simulink model "Controllo_Robusto"  (R2015a)
settings: Solver=ode3  StartTime=0.0  StopTime=40  FixedStep=1e-3  RelTol=1e-3
values from neighbouring files (symbols this model uses):
  alpha = in(85)    [fun_w.m]    (also in inicia_dinam.m = (BM-Bm)/(BM+Bm))
  BM = in(19)    [fun_w.m]    (also in inicia_dinam.m = norm(eval(B)))
  dif_t = in(9)    [Euler.m]    (also in rob_sic.m = 0.001)
  Kd = kd*eye(4)    [inicia_dinam.m]    (also in rob_sic.m = 50*eye(4))
  kd = in(18)    [fun_w.m]    (also in inicia_dinam.m = 100)
  Kp = kp*eye(4)    [inicia_dinam.m]    (also in rob_sic.m = 100*eye(4))
  kp = in(17)    [fun_w.m]    (also in inicia_dinam.m = 100)
  Q_vector = [Q1;Q2;Q3;Q4;Q5;Q6;Q7;Q8]    [inicia_dinam.m]
  QM = in(84)    [fun_w.m]    (also in inicia_dinam.m = norm(Q))
settings Model: Creator=TRIANOSAURIO  LastModifiedBy=TRIANOSAURIO
settings ConfigComp: CovMetricSettings=dw  CovHtmlReporting=on  CovSaveCumulativeToWorkspaceVar=on  CovSaveSingleToWorkspaceVar=on  CovExternalEMLEnable=off

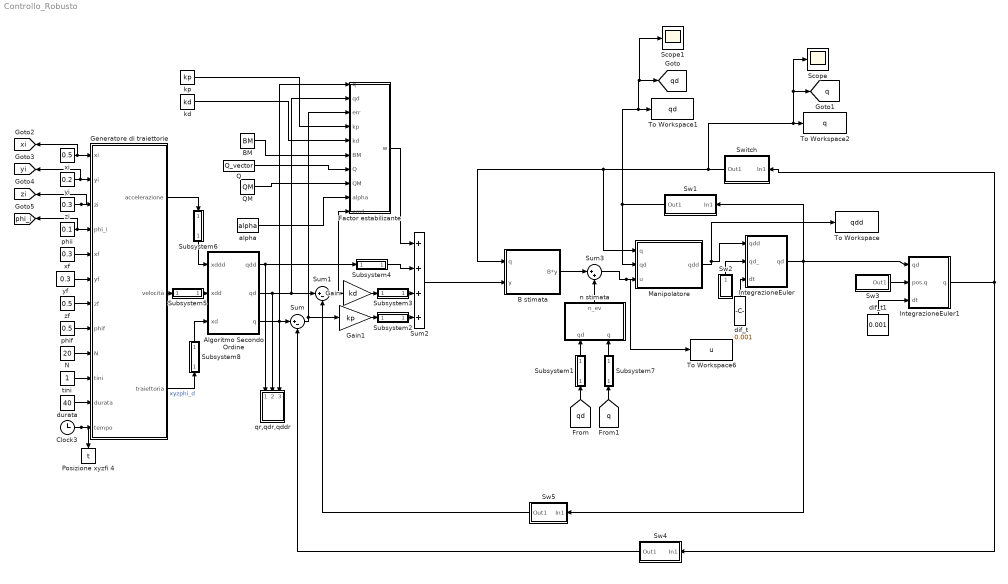
== system Controllo_Robusto ==
  Algoritmo Secondo Ordine : Subsystem
  B stimata : Subsystem
  "BM " : Constant  Value=BM
  Clock3 : Clock
  Factor estabilizante : Subsystem
  Gain : Gain  Gain=kd
  Gain1 : Gain  Gain=kp
  Generatore di traiettorie : Subsystem
  IntegrazioneEuler : Subsystem
  IntegrazioneEuler1 : Subsystem
  Manipolatore : Subsystem
  N : Constant  Value=20
  Posizione xyzfi 4 : ToWorkspace  VariableName=t  SampleTime=0.001
  Q : Constant  Value=Q_vector  VectorParams1D=off
  QM : Constant  Value=QM
  Scope : Scope
  Scope1 : Scope
  Subsystem1 : Subsystem
  Subsystem2 : Subsystem
  Subsystem3 : Subsystem
  Subsystem4 : Subsystem
  Subsystem5 : Subsystem
  Subsystem6 : Subsystem
  Subsystem7 : Subsystem
  Subsystem8 : Subsystem
  Sum : Sum  Inputs=|+-
  Sum1 : Sum  Inputs=|+-
  Sum2 : Sum  Inputs=++++
  Sum3 : Sum  Inputs=|++
  Sw1 : Subsystem
  Sw2 : Subsystem
  Sw3 : Subsystem
  Sw4 : Subsystem
  Sw5 : Subsystem
  Switch : Subsystem
  To Workspace : ToWorkspace  VariableName=qdd  SampleTime=-1
  To Workspace1 : ToWorkspace  VariableName=qd  SampleTime=-1
  To Workspace2 : ToWorkspace  VariableName=q  SampleTime=-1
  To Workspace6 : ToWorkspace  VariableName=u  SampleTime=-1
  alpha : Constant  Value=alpha
  dif_t : Constant  Value=0.001
  dif_t1 : Constant  Value=0.001
  durata : Constant  Value=40
  kd : Constant  Value=kd
  kp : Constant  Value=kp
  n stimata : Subsystem
  phif : Constant  Value=0.5
  phii : Constant  Value=0.1
  qr,qdr,qddr : Subsystem
  tini : Constant
  xf : Constant  Value=0.3
  xi : Constant  Value=0.5
  yf : Constant  Value=0.3
  yi : Constant  Value=0.2
  zf : Constant  Value=0.5
  zi : Constant  Value=0.3
  tag scope: phi_i=global, q=global, qd=global, xi=global, yi=global, zi=global
  wires:
  xi/1 -> [xi], Generatore di traiettorie/1(xi)
  yi/1 -> [yi], Generatore di traiettorie/2(yi)
  zi/1 -> [zi], Generatore di traiettorie/3(zi)
  phii/1 -> Generatore di traiettorie/4(phi_i), [phi_i]
  xf/1 -> Generatore di traiettorie/5(xf)
  yf/1 -> Generatore di traiettorie/6(yf)
  zf/1 -> Generatore di traiettorie/7(zf)
  phif/1 -> Generatore di traiettorie/8(phif)
  N/1 -> Generatore di traiettorie/9(N)
  tini/1 -> Generatore di traiettorie/10(tini)
  durata/1 -> Generatore di traiettorie/11(durata)
  Clock3/1 -> Posizione xyzfi 4/1, Generatore di traiettorie/12(tempo)
  Generatore di traiettorie/1(accelerazione) -> Subsystem6/1(In1)
  Algoritmo Secondo Ordine/3(q) -> Sum/1, Factor estabilizante/1(q), qr,qdr,qddr/3(In3)
  Sum/1 -> Factor estabilizante/3(err), Gain1/1
  Algoritmo Secondo Ordine/2(qd) -> Factor estabilizante/2(qd), Sum1/1, qr,qdr,qddr/2(In2)
  Sum1/1 -> Factor estabilizante/10(errd), Gain/1
  Algoritmo Secondo Ordine/1(qdd) -> qr,qdr,qddr/1(In1), Subsystem4/1(In1)
  Sum3/1 -> To Workspace6/1, Manipolatore/3(u)
  Manipolatore/1(qdd) -> IntegrazioneEuler/1(qdd), To Workspace/1
  Sum2/1 -> B stimata/2(y)
  B stimata/1("B*y ") -> Sum3/1
  kp/1 -> Factor estabilizante/4(kp)
  kd/1 -> Factor estabilizante/5(kd)
  "BM "/1 -> Factor estabilizante/6(BM)
  Q/1 -> Factor estabilizante/7(Q)
  QM/1 -> Factor estabilizante/8(QM)
  alpha/1 -> Factor estabilizante/9(alpha)
  Factor estabilizante/1(w) -> Sum2/1
  IntegrazioneEuler/1(qd) -> Sw5/1(In1), Sw1/1(In1), IntegrazioneEuler1/1(qd)
  IntegrazioneEuler1/1(q) -> Sw4/1(In1), Switch/1(In1)
  dif_t/1 -> IntegrazioneEuler/3(dt)
  dif_t1/1 -> IntegrazioneEuler1/3(dt)
  n stimata/1(n_ev) -> Sum3/2
  Generatore di traiettorie/3("traiettoria ") -> Subsystem8/1(In1)  "xyzphi_d"
  [qd] -> Subsystem1/1(In1)
  Subsystem1/1(Out1) -> n stimata/1(qd)
  [q] -> Subsystem7/1(In1)
  Subsystem7/1(Out1) -> n stimata/2(q)
  Gain1/1 -> Subsystem2/1(In1)
  Subsystem3/1(Out1) -> Sum2/3
  Gain/1 -> Subsystem3/1(In1)
  Subsystem2/1(Out1) -> Sum2/4
  Switch/1(Out1) -> Manipolatore/1(q), B stimata/1(q), Scope/1, [q], To Workspace2/1
  Sw1/1(Out1) -> Scope1/1, [qd], To Workspace1/1, Manipolatore/2(qd)
  Sw2/1(Out1) -> IntegrazioneEuler/2(qd_)
  Sw3/1(Out1) -> IntegrazioneEuler1/2(pos.q)
  Sw4/1(Out1) -> Sum/2
  Sw5/1(Out1) -> Sum1/2
  Subsystem4/1(Out1) -> Sum2/2
  Generatore di traiettorie/2(velocità) -> Subsystem5/1(In1)
  Subsystem5/1(Out1) -> Algoritmo Secondo Ordine/2(xdd)
  Subsystem6/1(Out1) -> Algoritmo Secondo Ordine/1(xddd)
  Subsystem8/1(Out1) -> Algoritmo Secondo Ordine/3(xd)

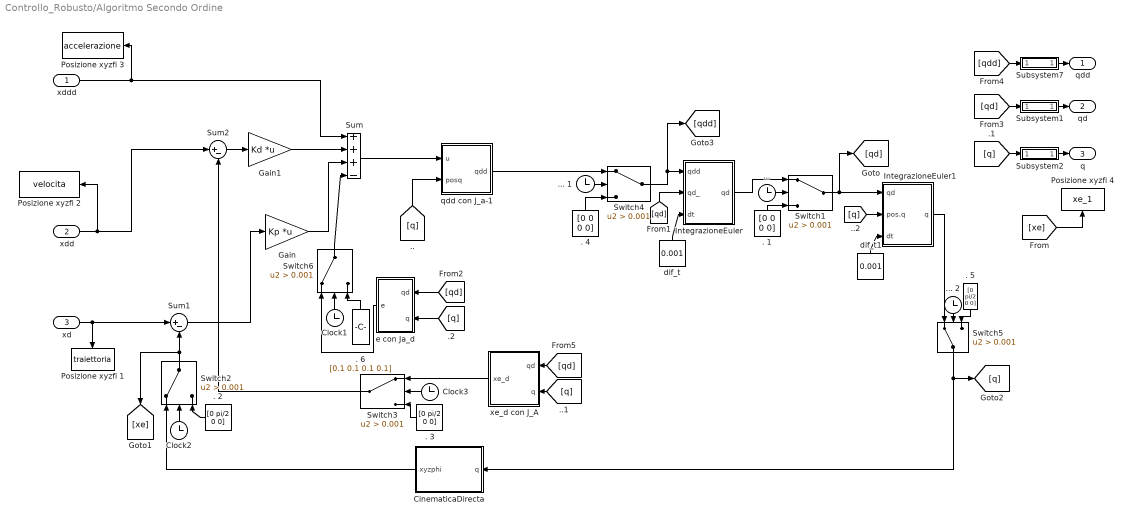
== system Controllo_Robusto/Algoritmo Secondo Ordine ==
  xddd : Inport
  xdd : Inport  Port=2
  xd : Inport  Port=3
  . 1 : Constant  Value=[0 0 0 0]
  . 2 : Constant  Value=[0 pi/2 0 0]
  . 3 : Constant  Value=[0 pi/2 0 0]
  . 4 : Constant  Value=[0 0 0 0]
  . 5 : Constant  Value=[0 pi/2 0 0]
  . 6 : Constant  Value=[0.1 0.1 0.1 0.1]
  "... " : Clock
  ... 1 : Clock
  ... 2 : Clock
  CinematicaDirecta : Subsystem
  Clock1 : Clock
  Clock2 : Clock
  Clock3 : Clock
  Gain : Gain  Gain=Kp  Multiplication=Matrix(K*u)
  Gain1 : Gain  Gain=Kd  Multiplication=Matrix(K*u)
  IntegrazioneEuler : Subsystem
  IntegrazioneEuler1 : Subsystem
  Posizione xyzfi 1 : ToWorkspace  VariableName=traiettoria  SampleTime=dif_t
  Posizione xyzfi 2 : ToWorkspace  VariableName=velocita  SampleTime=dif_t
  Posizione xyzfi 3 : ToWorkspace  VariableName=accelerazione  SampleTime=dif_t
  Posizione xyzfi 4 : ToWorkspace  VariableName=xe_1  SampleTime=dif_t
  Subsystem1 : Subsystem
  Subsystem2 : Subsystem
  Subsystem7 : Subsystem
  Sum : Sum  Inputs=+++-
  Sum1 : Sum  Inputs=|+-
  Sum2 : Sum  Inputs=|+-
  Switch{1..6} (6 alike) : Switch  Criteria=u2 > Threshold  Threshold=0.001
  dif_t : Constant  Value=0.001
  dif_t1 : Constant  Value=0.001
  e con Ja_d : Subsystem
  qdd con J_a-1 : Subsystem
  xe_d con J_A : Subsystem
  qdd : Outport
  qd : Outport  Port=2
  q : Outport  Port=3
  wires:
  Switch2/1 -> [xe], Sum1/2
  CinematicaDirecta/1(xyzphi) -> Switch2/1
  Clock2/1 -> Switch2/2
  . 2/1 -> Switch2/3
  dif_t/1 -> IntegrazioneEuler/3(dt)
  Sum1/1 -> Gain/1
  Sum/1 -> qdd con J_a-1/1(u)
  [q] -> qdd con J_a-1/2(posq)
  [qd] -> IntegrazioneEuler/2(qd_)
  xd/1 -> Sum1/1, Posizione xyzfi 1/1
  xdd/1 -> Posizione xyzfi 2/1, Sum2/1
  [q] -> xe_d con J_A/2(q)
  Gain/1 -> Sum/3
  Sum2/1 -> Gain1/1
  Gain1/1 -> Sum/2
  xddd/1 -> Posizione xyzfi 3/1, Sum/1
  Clock3/1 -> Switch3/2
  . 3/1 -> Switch3/3
  xe_d con J_A/1(xe_d) -> Switch3/1
  Switch3/1 -> Sum2/2
  dif_t1/1 -> IntegrazioneEuler1/3(dt)
  [q] -> e con Ja_d/2(q)
  [xe] -> Posizione xyzfi 4/1
  IntegrazioneEuler1/1(q) -> Switch5/1
  . 5/1 -> Switch5/3
  ... 2/1 -> Switch5/2
  Switch5/1 -> [q], CinematicaDirecta/1(q)
  [q] -> IntegrazioneEuler1/2(pos.q)
  IntegrazioneEuler/1(qd) -> Switch1/1
  . 1/1 -> Switch1/3
  "... "/1 -> Switch1/2
  Switch1/1 -> IntegrazioneEuler1/1(qd), [qd]
  [qd] -> e con Ja_d/1(qd)
  qdd con J_a-1/1(qdd) -> Switch4/1
  . 4/1 -> Switch4/3
  ... 1/1 -> Switch4/2
  Switch4/1 -> [qdd], IntegrazioneEuler/1(qdd)
  [qd] -> xe_d con J_A/1(qd)
  Clock1/1 -> Switch6/2
  . 6/1 -> Switch6/3
  e con Ja_d/1(e) -> Switch6/1
  Switch6/1 -> Sum/4
  [qdd] -> Subsystem7/1(In1)
  [qd] -> Subsystem1/1(In1)
  Subsystem1/1(Out1) -> qd/1
  [q] -> Subsystem2/1(In1)
  Subsystem2/1(Out1) -> q/1
  Subsystem7/1(Out1) -> qdd/1

== system Controllo_Robusto/B stimata ==
  q : Inport
  y : Inport  Port=2
  "B_stimata " : MATLABFcn  MATLABFcn=fun_B
  Mux1 : Mux  Inputs=2
  "B*y " : Outport
  wires:
  "B_stimata "/1 -> "B*y "/1
  Mux1/1 -> "B_stimata "/1
  q/1 -> Mux1/2
  y/1 -> Mux1/1

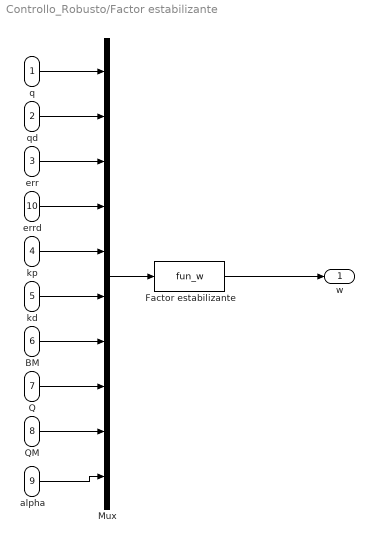
== system Controllo_Robusto/Factor estabilizante ==
  q : Inport
  qd : Inport  Port=2
  err : Inport  Port=3
  kp : Inport  Port=4
  kd : Inport  Port=5
  BM : Inport  Port=6
  Q : Inport  Port=7
  QM : Inport  Port=8
  alpha : Inport  Port=9
  errd : Inport  Port=10
  Factor estabilizante : MATLABFcn  MATLABFcn=fun_w  OutputDimensions=4
  Mux : Mux  Inputs=10
  w : Outport
  wires:
  Mux/1 -> Factor estabilizante/1
  qd/1 -> Mux/2
  q/1 -> Mux/1
  err/1 -> Mux/3
  errd/1 -> Mux/4
  kp/1 -> Mux/5
  kd/1 -> Mux/6
  BM/1 -> Mux/7
  Q/1 -> Mux/8
  QM/1 -> Mux/9
  alpha/1 -> Mux/10
  Factor estabilizante/1 -> w/1

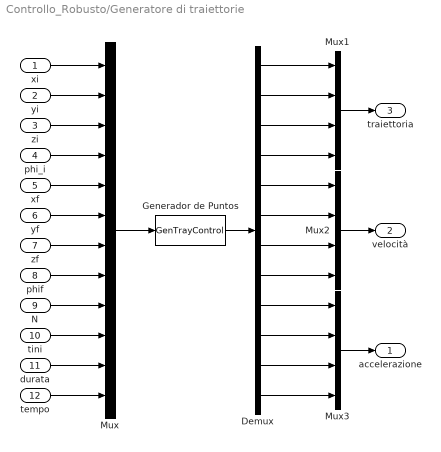
== system Controllo_Robusto/Generatore di traiettorie ==
  xi : Inport
  yi : Inport  Port=2
  zi : Inport  Port=3
  phi_i : Inport  Port=4
  xf : Inport  Port=5
  yf : Inport  Port=6
  zf : Inport  Port=7
  phif : Inport  Port=8
  N : Inport  Port=9
  tini : Inport  Port=10
  durata : Inport  Port=11
  tempo : Inport  Port=12
  Demux : Demux  Outputs=12
  Generador de Puntos : MATLABFcn  MATLABFcn=GenTrayControl  OutputDimensions=12
  Mux : Mux  Inputs=12
  Mux1 : Mux
  Mux2 : Mux
  Mux3 : Mux
  accelerazione : Outport
  velocità : Outport  Port=2
  "traiettoria " : Outport  Port=3
  wires:
  Mux/1 -> Generador de Puntos/1
  xi/1 -> Mux/1
  yi/1 -> Mux/2
  zi/1 -> Mux/3
  phi_i/1 -> Mux/4
  xf/1 -> Mux/5
  yf/1 -> Mux/6
  zf/1 -> Mux/7
  phif/1 -> Mux/8
  N/1 -> Mux/9
  tini/1 -> Mux/10
  durata/1 -> Mux/11
  tempo/1 -> Mux/12
  Generador de Puntos/1 -> Demux/1
  Mux1/1 -> "traiettoria "/1
  Mux2/1 -> velocità/1
  Mux3/1 -> accelerazione/1
  Demux/12 -> Mux3/4
  Demux/11 -> Mux3/3
  Demux/10 -> Mux3/2
  Demux/9 -> Mux3/1
  Demux/8 -> Mux2/4
  Demux/7 -> Mux2/3
  Demux/6 -> Mux2/2
  Demux/5 -> Mux2/1
  Demux/4 -> Mux1/4
  Demux/1 -> Mux1/1
  Demux/2 -> Mux1/2
  Demux/3 -> Mux1/3

== system Controllo_Robusto/IntegrazioneEuler ==
  qdd : Inport
  qd_ : Inport  Port=2
  dt : Inport  Port=3
  Euler : MATLABFcn  MATLABFcn=Euler  OutputDimensions=4
  Mux2 : Mux  Inputs=3
  Subsystem4 : Subsystem
  qd : Outport
  wires:
  Euler/1 -> Subsystem4/1(In1)
  qdd/1 -> Mux2/1
  Mux2/1 -> Euler/1
  qd_/1 -> Mux2/2
  dt/1 -> Mux2/3
  Subsystem4/1(Out1) -> qd/1

== system Controllo_Robusto/IntegrazioneEuler1 ==
  qd : Inport
  pos.q : Inport  Port=2
  dt : Inport  Port=3
  Euler : MATLABFcn  MATLABFcn=Euler  OutputDimensions=4
  Mux2 : Mux  Inputs=3
  Subsystem4 : Subsystem
  q : Outport
  wires:
  dt/1 -> Mux2/3
  pos.q/1 -> Mux2/2
  Mux2/1 -> Euler/1
  qd/1 -> Mux2/1
  Euler/1 -> Subsystem4/1(In1)
  Subsystem4/1(Out1) -> q/1

== system Controllo_Robusto/Manipolatore ==
  q : Inport
  qd : Inport  Port=2
  u : Inport  Port=3
  Manipolatore : MATLABFcn  MATLABFcn=modelo_dinam  OutputDimensions=4
  Mux3 : Mux
  Subsystem4 : Subsystem
  qdd : Outport
  wires:
  Mux3/1 -> Manipolatore/1
  u/1 -> Mux3/1
  q/1 -> Mux3/2
  qd/1 -> Mux3/3
  Manipolatore/1 -> Subsystem4/1(In1)
  Subsystem4/1(Out1) -> Mux3/4, qdd/1

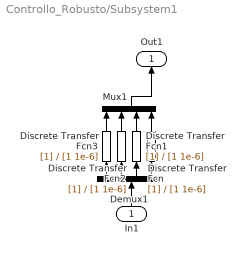
== system Controllo_Robusto/Subsystem1 ==
  In1 : Inport
  Demux1 : Demux
  Discrete Transfer Fcn{,1..3} (4 alike) : DiscreteTransferFcn  Denominator=[1 1e-6]  SampleTime=0.001
  Mux1 : Mux
  Out1 : Outport
  wires:
  In1/1 -> Demux1/1
  Mux1/1 -> Out1/1
  Discrete Transfer Fcn/1 -> Mux1/4
  Demux1/4 -> Discrete Transfer Fcn/1
  Discrete Transfer Fcn1/1 -> Mux1/3
  Demux1/3 -> Discrete Transfer Fcn1/1
  Discrete Transfer Fcn2/1 -> Mux1/2
  Demux1/2 -> Discrete Transfer Fcn2/1
  Discrete Transfer Fcn3/1 -> Mux1/1
  Demux1/1 -> Discrete Transfer Fcn3/1

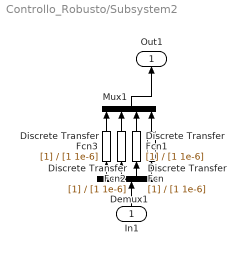
== system Controllo_Robusto/Subsystem2 ==
  In1 : Inport
  Demux1 : Demux
  Discrete Transfer Fcn{,1..3} (4 alike) : DiscreteTransferFcn  Denominator=[1 1e-6]  SampleTime=0.001
  Mux1 : Mux
  Out1 : Outport
  wires:
  In1/1 -> Demux1/1
  Mux1/1 -> Out1/1
  Discrete Transfer Fcn/1 -> Mux1/4
  Demux1/4 -> Discrete Transfer Fcn/1
  Discrete Transfer Fcn1/1 -> Mux1/3
  Demux1/3 -> Discrete Transfer Fcn1/1
  Discrete Transfer Fcn2/1 -> Mux1/2
  Demux1/2 -> Discrete Transfer Fcn2/1
  Discrete Transfer Fcn3/1 -> Mux1/1
  Demux1/1 -> Discrete Transfer Fcn3/1

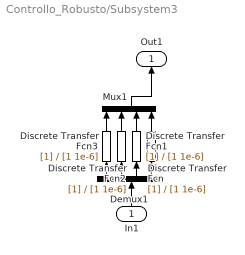
== system Controllo_Robusto/Subsystem3 ==
  In1 : Inport
  Demux1 : Demux
  Discrete Transfer Fcn{,1..3} (4 alike) : DiscreteTransferFcn  Denominator=[1 1e-6]  SampleTime=0.001
  Mux1 : Mux
  Out1 : Outport
  wires:
  Demux1/1 -> Discrete Transfer Fcn3/1
  Discrete Transfer Fcn3/1 -> Mux1/1
  Demux1/2 -> Discrete Transfer Fcn2/1
  Discrete Transfer Fcn2/1 -> Mux1/2
  Demux1/3 -> Discrete Transfer Fcn1/1
  Discrete Transfer Fcn1/1 -> Mux1/3
  Demux1/4 -> Discrete Transfer Fcn/1
  Discrete Transfer Fcn/1 -> Mux1/4
  Mux1/1 -> Out1/1
  In1/1 -> Demux1/1

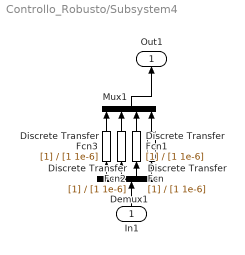
== system Controllo_Robusto/Subsystem4 ==
  In1 : Inport
  Demux1 : Demux
  Discrete Transfer Fcn{,1..3} (4 alike) : DiscreteTransferFcn  Denominator=[1 1e-6]  SampleTime=0.001
  Mux1 : Mux
  Out1 : Outport
  wires:
  In1/1 -> Demux1/1
  Mux1/1 -> Out1/1
  Discrete Transfer Fcn/1 -> Mux1/4
  Demux1/4 -> Discrete Transfer Fcn/1
  Discrete Transfer Fcn1/1 -> Mux1/3
  Demux1/3 -> Discrete Transfer Fcn1/1
  Discrete Transfer Fcn2/1 -> Mux1/2
  Demux1/2 -> Discrete Transfer Fcn2/1
  Discrete Transfer Fcn3/1 -> Mux1/1
  Demux1/1 -> Discrete Transfer Fcn3/1

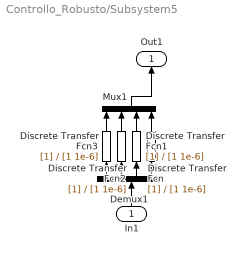
== system Controllo_Robusto/Subsystem5 ==
  In1 : Inport
  Demux1 : Demux
  Discrete Transfer Fcn{,1..3} (4 alike) : DiscreteTransferFcn  Denominator=[1 1e-6]  SampleTime=0.001
  Mux1 : Mux
  Out1 : Outport
  wires:
  In1/1 -> Demux1/1
  Mux1/1 -> Out1/1
  Discrete Transfer Fcn/1 -> Mux1/4
  Demux1/4 -> Discrete Transfer Fcn/1
  Discrete Transfer Fcn1/1 -> Mux1/3
  Demux1/3 -> Discrete Transfer Fcn1/1
  Discrete Transfer Fcn2/1 -> Mux1/2
  Demux1/2 -> Discrete Transfer Fcn2/1
  Discrete Transfer Fcn3/1 -> Mux1/1
  Demux1/1 -> Discrete Transfer Fcn3/1

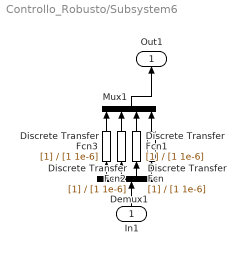
== system Controllo_Robusto/Subsystem6 ==
  In1 : Inport
  Demux1 : Demux
  Discrete Transfer Fcn{,1..3} (4 alike) : DiscreteTransferFcn  Denominator=[1 1e-6]  SampleTime=0.001
  Mux1 : Mux
  Out1 : Outport
  wires:
  Demux1/1 -> Discrete Transfer Fcn3/1
  Discrete Transfer Fcn3/1 -> Mux1/1
  Demux1/2 -> Discrete Transfer Fcn2/1
  Discrete Transfer Fcn2/1 -> Mux1/2
  Demux1/3 -> Discrete Transfer Fcn1/1
  Discrete Transfer Fcn1/1 -> Mux1/3
  Demux1/4 -> Discrete Transfer Fcn/1
  Discrete Transfer Fcn/1 -> Mux1/4
  Mux1/1 -> Out1/1
  In1/1 -> Demux1/1

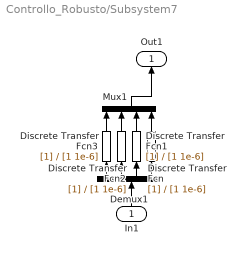
== system Controllo_Robusto/Subsystem7 ==
  In1 : Inport
  Demux1 : Demux
  Discrete Transfer Fcn{,1..3} (4 alike) : DiscreteTransferFcn  Denominator=[1 1e-6]  SampleTime=0.001
  Mux1 : Mux
  Out1 : Outport
  wires:
  In1/1 -> Demux1/1
  Mux1/1 -> Out1/1
  Discrete Transfer Fcn/1 -> Mux1/4
  Demux1/4 -> Discrete Transfer Fcn/1
  Discrete Transfer Fcn1/1 -> Mux1/3
  Demux1/3 -> Discrete Transfer Fcn1/1
  Discrete Transfer Fcn2/1 -> Mux1/2
  Demux1/2 -> Discrete Transfer Fcn2/1
  Discrete Transfer Fcn3/1 -> Mux1/1
  Demux1/1 -> Discrete Transfer Fcn3/1

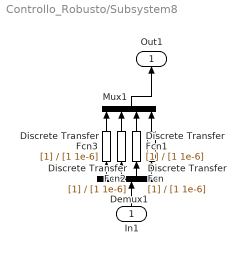
== system Controllo_Robusto/Subsystem8 ==
  In1 : Inport
  Demux1 : Demux
  Discrete Transfer Fcn{,1..3} (4 alike) : DiscreteTransferFcn  Denominator=[1 1e-6]  SampleTime=0.001
  Mux1 : Mux
  Out1 : Outport
  wires:
  In1/1 -> Demux1/1
  Mux1/1 -> Out1/1
  Discrete Transfer Fcn/1 -> Mux1/4
  Demux1/4 -> Discrete Transfer Fcn/1
  Discrete Transfer Fcn1/1 -> Mux1/3
  Demux1/3 -> Discrete Transfer Fcn1/1
  Discrete Transfer Fcn2/1 -> Mux1/2
  Demux1/2 -> Discrete Transfer Fcn2/1
  Discrete Transfer Fcn3/1 -> Mux1/1
  Demux1/1 -> Discrete Transfer Fcn3/1

== system Controllo_Robusto/Sw1 ==
  In1 : Inport
  . 5 : Constant  Value=[0 0 0 0]
  Clock6 : Clock
  Subsystem9 : Subsystem
  Switch5 : Switch  Criteria=u2 > Threshold  Threshold=0.001
  Out1 : Outport
  wires:
  In1/1 -> Subsystem9/1(In1)
  Subsystem9/1(Out1) -> Switch5/1
  Switch5/1 -> Out1/1
  . 5/1 -> Switch5/3
  Clock6/1 -> Switch5/2

== system Controllo_Robusto/Sw2 ==
  . 7 : Constant  Value=[0 pi/2 0 0]
  "... " : Clock
  Switch7 : Switch  Criteria=u2 > Threshold  Threshold=0.001
  Out1 : Outport
  wires:
  "... "/1 -> Switch7/2
  . 7/1 -> Switch7/3
  [qd] -> Switch7/1
  Switch7/1 -> Out1/1

== system Controllo_Robusto/Sw3 ==
  ... 1 : Clock
  Switch8 : Switch  Criteria=u2 > Threshold  Threshold=0.001
  dif_t : Constant  Value=[0 pi/2 0 0]
  Out1 : Outport
  wires:
  [q] -> Switch8/1
  dif_t/1 -> Switch8/3
  Switch8/1 -> Out1/1
  ... 1/1 -> Switch8/2

== system Controllo_Robusto/Sw4 ==
  In1 : Inport
  Clock1 : Clock
  Switch3 : Switch  Criteria=u2 > Threshold  Threshold=0.001
  dif_t : Constant  Value=[0 pi/2 0 0]
  Out1 : Outport
  wires:
  In1/1 -> Switch3/1
  dif_t/1 -> Switch3/3
  Clock1/1 -> Switch3/2
  Switch3/1 -> Out1/1

== system Controllo_Robusto/Sw5 ==
  In1 : Inport
  . 1 : Constant  Value=[0 0 0 0]
  Clock2 : Clock
  Subsystem4 : Subsystem
  Switch1 : Switch  Criteria=u2 > Threshold  Threshold=0.001
  Out1 : Outport
  wires:
  In1/1 -> Subsystem4/1(In1)
  Clock2/1 -> Switch1/2
  . 1/1 -> Switch1/3
  Switch1/1 -> Out1/1
  Subsystem4/1(Out1) -> Switch1/1

== system Controllo_Robusto/Switch ==
  In1 : Inport
  Clock7 : Clock
  Subsystem8 : Subsystem
  Switch6 : Switch  Criteria=u2 > Threshold  Threshold=0.001
  dif_t : Constant  Value=[0 pi/2 0 0]
  Out1 : Outport
  wires:
  In1/1 -> Subsystem8/1(In1)
  Subsystem8/1(Out1) -> Switch6/1
  Clock7/1 -> Switch6/2
  Switch6/1 -> Out1/1
  dif_t/1 -> Switch6/3

== system Controllo_Robusto/n stimata ==
  qd : Inport
  q : Inport  Port=2
  Mux2 : Mux  Inputs=2
  "n_stimata " : MATLABFcn  MATLABFcn=fun_n  OutputDimensions=4
  n_ev : Outport
  wires:
  Mux2/1 -> "n_stimata "/1
  q/1 -> Mux2/1
  qd/1 -> Mux2/2
  "n_stimata "/1 -> n_ev/1

== system Controllo_Robusto/qr,qdr,qddr ==
  In1 : Inport
  In2 : Inport  Port=2
  In3 : Inport  Port=3
  To Workspace3 : ToWorkspace  VariableName=qr  SampleTime=-1
  To Workspace4 : ToWorkspace  VariableName=qdr  SampleTime=-1
  To Workspace5 : ToWorkspace  VariableName=qddr  SampleTime=-1
  wires:
  In3/1 -> To Workspace3/1
  In2/1 -> To Workspace4/1
  In1/1 -> To Workspace5/1

== system Controllo_Robusto/Algoritmo Secondo Ordine/CinematicaDirecta ==
  q : Inport
  Interpreted MATLAB Function : MATLABFcn  MATLABFcn=CinematicaDirecta
  xyzphi : Outport
  wires:
  q/1 -> Interpreted MATLAB Function/1
  Interpreted MATLAB Function/1 -> xyzphi/1

== system Controllo_Robusto/Algoritmo Secondo Ordine/IntegrazioneEuler ==
  qdd : Inport
  qd_ : Inport  Port=2
  dt : Inport  Port=3
  Euler : MATLABFcn  MATLABFcn=Euler
  Mux2 : Mux  Inputs=3
  qd : Outport
  wires:
  Euler/1 -> qd/1
  qdd/1 -> Mux2/1
  Mux2/1 -> Euler/1
  qd_/1 -> Mux2/2
  dt/1 -> Mux2/3

== system Controllo_Robusto/Algoritmo Secondo Ordine/IntegrazioneEuler1 ==
  qd : Inport
  pos.q : Inport  Port=2
  dt : Inport  Port=3
  Euler : MATLABFcn  MATLABFcn=Euler
  Mux2 : Mux  Inputs=3
  q : Outport
  wires:
  dt/1 -> Mux2/3
  pos.q/1 -> Mux2/2
  Mux2/1 -> Euler/1
  qd/1 -> Mux2/1
  Euler/1 -> q/1

== system Controllo_Robusto/Algoritmo Secondo Ordine/Subsystem1 ==
  In1 : Inport
  Demux1 : Demux
  Discrete Transfer Fcn{,1..3} (4 alike) : DiscreteTransferFcn  Denominator=[1 1e-6]  SampleTime=0.001
  Mux1 : Mux
  Out1 : Outport
  wires:
  Demux1/1 -> Discrete Transfer Fcn3/1
  Discrete Transfer Fcn3/1 -> Mux1/1
  Demux1/2 -> Discrete Transfer Fcn2/1
  Discrete Transfer Fcn2/1 -> Mux1/2
  Demux1/3 -> Discrete Transfer Fcn1/1
  Discrete Transfer Fcn1/1 -> Mux1/3
  Demux1/4 -> Discrete Transfer Fcn/1
  Discrete Transfer Fcn/1 -> Mux1/4
  Mux1/1 -> Out1/1
  In1/1 -> Demux1/1

== system Controllo_Robusto/Algoritmo Secondo Ordine/Subsystem2 ==
  In1 : Inport
  Demux1 : Demux
  Discrete Transfer Fcn{,1..3} (4 alike) : DiscreteTransferFcn  Denominator=[1 1e-6]  SampleTime=0.001
  Mux1 : Mux
  Out1 : Outport
  wires:
  In1/1 -> Demux1/1
  Mux1/1 -> Out1/1
  Discrete Transfer Fcn/1 -> Mux1/4
  Demux1/4 -> Discrete Transfer Fcn/1
  Discrete Transfer Fcn1/1 -> Mux1/3
  Demux1/3 -> Discrete Transfer Fcn1/1
  Discrete Transfer Fcn2/1 -> Mux1/2
  Demux1/2 -> Discrete Transfer Fcn2/1
  Discrete Transfer Fcn3/1 -> Mux1/1
  Demux1/1 -> Discrete Transfer Fcn3/1

== system Controllo_Robusto/Algoritmo Secondo Ordine/Subsystem7 ==
  In1 : Inport
  Demux1 : Demux
  Discrete Transfer Fcn{,1..3} (4 alike) : DiscreteTransferFcn  Denominator=[1 1e-6]  SampleTime=0.001
  Mux1 : Mux
  Out1 : Outport
  wires:
  In1/1 -> Demux1/1
  Mux1/1 -> Out1/1
  Discrete Transfer Fcn/1 -> Mux1/4
  Demux1/4 -> Discrete Transfer Fcn/1
  Discrete Transfer Fcn1/1 -> Mux1/3
  Demux1/3 -> Discrete Transfer Fcn1/1
  Discrete Transfer Fcn2/1 -> Mux1/2
  Demux1/2 -> Discrete Transfer Fcn2/1
  Discrete Transfer Fcn3/1 -> Mux1/1
  Demux1/1 -> Discrete Transfer Fcn3/1

== system Controllo_Robusto/Algoritmo Secondo Ordine/e con Ja_d ==
  qd : Inport
  q : Inport  Port=2
  JacobianaDerivada : MATLABFcn  MATLABFcn=JacobianaDerivada
  Mux2 : Mux  Inputs=2
  Subsystem4 : Subsystem
  e : Outport
  wires:
  q/1 -> Mux2/2
  JacobianaDerivada/1 -> Subsystem4/1(In1)
  qd/1 -> Mux2/1
  Mux2/1 -> JacobianaDerivada/1
  Subsystem4/1(Out1) -> e/1

== system Controllo_Robusto/Algoritmo Secondo Ordine/qdd con J_a-1 ==
  u : Inport
  posq : Inport  Port=2
  Mux2 : Mux  Inputs=2
  qd_mediante_Ja-1 : MATLABFcn  MATLABFcn=JacobianaNumerica
  qdd : Outport
  wires:
  qd_mediante_Ja-1/1 -> qdd/1
  Mux2/1 -> qd_mediante_Ja-1/1
  u/1 -> Mux2/1
  posq/1 -> Mux2/2

== system Controllo_Robusto/Algoritmo Secondo Ordine/xe_d con J_A ==
  qd : Inport
  q : Inport  Port=2
  Mux2 : Mux  Inputs=2
  "xe^{.}" : MATLABFcn  MATLABFcn=JacobianaAnalitica
  xe_d : Outport
  wires:
  q/1 -> Mux2/2
  Mux2/1 -> "xe^{.}"/1
  qd/1 -> Mux2/1
  "xe^{.}"/1 -> xe_d/1

== system Controllo_Robusto/IntegrazioneEuler/Subsystem4 ==
  In1 : Inport
  Demux1 : Demux
  Discrete Transfer Fcn{,1..3} (4 alike) : DiscreteTransferFcn  Denominator=[1 1e-6]  SampleTime=0.001
  Mux1 : Mux
  Out1 : Outport
  wires:
  In1/1 -> Demux1/1
  Mux1/1 -> Out1/1
  Discrete Transfer Fcn/1 -> Mux1/4
  Demux1/4 -> Discrete Transfer Fcn/1
  Discrete Transfer Fcn1/1 -> Mux1/3
  Demux1/3 -> Discrete Transfer Fcn1/1
  Discrete Transfer Fcn2/1 -> Mux1/2
  Demux1/2 -> Discrete Transfer Fcn2/1
  Discrete Transfer Fcn3/1 -> Mux1/1
  Demux1/1 -> Discrete Transfer Fcn3/1

== system Controllo_Robusto/IntegrazioneEuler1/Subsystem4 ==
  In1 : Inport
  Demux1 : Demux
  Discrete Transfer Fcn{,1..3} (4 alike) : DiscreteTransferFcn  Denominator=[1 1e-6]  SampleTime=0.001
  Mux1 : Mux
  Out1 : Outport
  wires:
  In1/1 -> Demux1/1
  Mux1/1 -> Out1/1
  Discrete Transfer Fcn/1 -> Mux1/4
  Demux1/4 -> Discrete Transfer Fcn/1
  Discrete Transfer Fcn1/1 -> Mux1/3
  Demux1/3 -> Discrete Transfer Fcn1/1
  Discrete Transfer Fcn2/1 -> Mux1/2
  Demux1/2 -> Discrete Transfer Fcn2/1
  Discrete Transfer Fcn3/1 -> Mux1/1
  Demux1/1 -> Discrete Transfer Fcn3/1

== system Controllo_Robusto/Manipolatore/Subsystem4 ==
  In1 : Inport
  Demux1 : Demux
  Discrete Transfer Fcn{,1..3} (4 alike) : DiscreteTransferFcn  Denominator=[1 1e-6]  SampleTime=0.001
  Mux1 : Mux
  Out1 : Outport
  wires:
  In1/1 -> Demux1/1
  Mux1/1 -> Out1/1
  Discrete Transfer Fcn/1 -> Mux1/4
  Demux1/4 -> Discrete Transfer Fcn/1
  Discrete Transfer Fcn1/1 -> Mux1/3
  Demux1/3 -> Discrete Transfer Fcn1/1
  Discrete Transfer Fcn2/1 -> Mux1/2
  Demux1/2 -> Discrete Transfer Fcn2/1
  Discrete Transfer Fcn3/1 -> Mux1/1
  Demux1/1 -> Discrete Transfer Fcn3/1

== system Controllo_Robusto/Sw1/Subsystem9 ==
  In1 : Inport
  Demux1 : Demux
  Discrete Transfer Fcn{,1..3} (4 alike) : DiscreteTransferFcn  Denominator=[1 1e-6]  SampleTime=0.001
  Mux1 : Mux
  Out1 : Outport
  wires:
  In1/1 -> Demux1/1
  Mux1/1 -> Out1/1
  Discrete Transfer Fcn/1 -> Mux1/4
  Demux1/4 -> Discrete Transfer Fcn/1
  Discrete Transfer Fcn1/1 -> Mux1/3
  Demux1/3 -> Discrete Transfer Fcn1/1
  Discrete Transfer Fcn2/1 -> Mux1/2
  Demux1/2 -> Discrete Transfer Fcn2/1
  Discrete Transfer Fcn3/1 -> Mux1/1
  Demux1/1 -> Discrete Transfer Fcn3/1

== system Controllo_Robusto/Sw5/Subsystem4 ==
  In1 : Inport
  Demux1 : Demux
  Discrete Transfer Fcn{,1..3} (4 alike) : DiscreteTransferFcn  Denominator=[1 1e-6]  SampleTime=0.001
  Mux1 : Mux
  Out1 : Outport
  wires:
  In1/1 -> Demux1/1
  Mux1/1 -> Out1/1
  Discrete Transfer Fcn/1 -> Mux1/4
  Demux1/4 -> Discrete Transfer Fcn/1
  Discrete Transfer Fcn1/1 -> Mux1/3
  Demux1/3 -> Discrete Transfer Fcn1/1
  Discrete Transfer Fcn2/1 -> Mux1/2
  Demux1/2 -> Discrete Transfer Fcn2/1
  Discrete Transfer Fcn3/1 -> Mux1/1
  Demux1/1 -> Discrete Transfer Fcn3/1

== system Controllo_Robusto/Switch/Subsystem8 ==
  In1 : Inport
  Demux1 : Demux
  Discrete Transfer Fcn{,1..3} (4 alike) : DiscreteTransferFcn  Denominator=[1 1e-6]  SampleTime=0.001
  Mux1 : Mux
  Out1 : Outport
  wires:
  In1/1 -> Demux1/1
  Mux1/1 -> Out1/1
  Discrete Transfer Fcn/1 -> Mux1/4
  Demux1/4 -> Discrete Transfer Fcn/1
  Discrete Transfer Fcn1/1 -> Mux1/3
  Demux1/3 -> Discrete Transfer Fcn1/1
  Discrete Transfer Fcn2/1 -> Mux1/2
  Demux1/2 -> Discrete Transfer Fcn2/1
  Discrete Transfer Fcn3/1 -> Mux1/1
  Demux1/1 -> Discrete Transfer Fcn3/1

== system Controllo_Robusto/Algoritmo Secondo Ordine/e con Ja_d/Subsystem4 ==
  In1 : Inport
  Demux1 : Demux
  Discrete Transfer Fcn{,1..3} (4 alike) : DiscreteTransferFcn  Denominator=[1 1e-6]  SampleTime=0.001
  Mux1 : Mux
  Out1 : Outport
  wires:
  In1/1 -> Demux1/1
  Mux1/1 -> Out1/1
  Discrete Transfer Fcn/1 -> Mux1/4
  Demux1/4 -> Discrete Transfer Fcn/1
  Discrete Transfer Fcn1/1 -> Mux1/3
  Demux1/3 -> Discrete Transfer Fcn1/1
  Discrete Transfer Fcn2/1 -> Mux1/2
  Demux1/2 -> Discrete Transfer Fcn2/1
  Discrete Transfer Fcn3/1 -> Mux1/1
  Demux1/1 -> Discrete Transfer Fcn3/1
